simulink model "Ex1"  (R2019a)
settings: Solver=VariableStepAuto  StartTime=0.0  StopTime=10.0  RelTol=1e-3
values from neighbouring files (symbols this model uses):
  K1 = 1    [value0.m]    (also in value1.m = 0.5)
  K2 = 2    [value0.m]    (also in value1.m = 1)
  K3 = 3    [value0.m]    (also in value1.m = 2)
  T = 1    [value0.m]    (also in value1.m = 2)
settings Model: Creator=Takumi SHIOTA  LastModifiedBy=Takumi SHIOTA

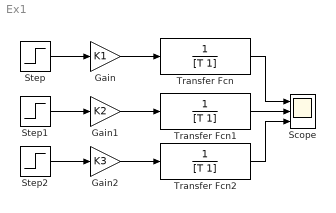
== system Ex1 ==
  Gain : Gain  Gain=K1
  Gain1 : Gain  Gain=K2
  Gain2 : Gain  Gain=K3
  Scope : Scope  NumInputPorts=3
  Step : Step  Time=0  SampleTime=0
  Step1 : Step  Time=0  SampleTime=0
  Step2 : Step  Time=0  SampleTime=0
  Transfer Fcn : TransferFcn  Denominator=[T 1]
  Transfer Fcn1 : TransferFcn  Denominator=[T 1]
  Transfer Fcn2 : TransferFcn  Denominator=[T 1]
  wires:
  Gain1/1 -> Transfer Fcn1/1
  Transfer Fcn/1 -> Scope/1
  Step/1 -> Gain/1
  Transfer Fcn2/1 -> Scope/3
  Gain2/1 -> Transfer Fcn2/1
  Step2/1 -> Gain2/1
  Gain/1 -> Transfer Fcn/1
  Step1/1 -> Gain1/1
  Transfer Fcn1/1 -> Scope/2
